simulink model "BatterySOHEstimation"  (R2024b)
settings: Solver=VariableStepAuto  StartTime=0.0  StopTime=3600  FixedStep=Ts  RelTol=1e-3  EnableMultiTasking=on
PreLoadFcn:
  | BatterySOHEstimationData;
values from neighbouring files (symbols this model uses):
  R = 0.05    [BatterySOHEstimationData.m]
  R00 = 0.008    [BatterySOHEstimationData.m]
  R0_mat = [.0117, .0085, .009; .011, .0085, .009;     .0114, .0087, .0092; .0107, .0082, .0088; .0107, .0083, .0091;     .0113, .0085, .0089; .0116, .0085, .0089]    [BatterySOHEstimationData.m]
  SOC0 = 0.65    [BatterySOHEstimationData.m]
  Ts = 1    [BatterySOHEstimationData.m]
undefined symbols (not defined in the file or in its folder): battery_builder_rtmsupport, gcbh
libraries: mBatteryPack_series_lib x414, mBatteryPack_lib x72, fl_lib x46, nesl_utility x22, BatteryEstimators x12, simulink x11, dspstat3 x9, PouchBatteryPack_lib x6, BatteryCurrentManagement x2, batteryecm_lib x1, SingleCellBatteryPack_lib x1
(part 1 of 26)
CloseFcn:
  | try
  |     close(h1_BatterySOHEstimation)
  | catch
  | end
  | 
  | clear h1_BatterySOHEstimation
  | 
  | clear BatterySOHEstimationSimlog
  | clear BatterySOHEstimationLogsout
  | 
  | clear AH SOC_vec T_vec R0_mat R1_mat tau1_mat
  | clear V0_mat Q R P0 initialSOC SOC0 R00 Ts
  | clear cell_area h_conv thermal_mass
Description:
  | Battery State-of-Health Estimation
settings Model: SimulationMode=accelerator  Creator=The MathWorks, Inc.  LastModifiedBy=marco
settings SolverCC: AlgebraicLoopSolver=TrustRegion  AutoInsertRateTranBlk=on  MaxZcPerStep=1
settings DataIOCC: MaxDataPoints=370000  ReturnWorkspaceOutputs=off  SignalLoggingName=BatterySOHEstimationLogsout
settings OptimizationCC: ReuseModelBlockBuffer=off  LifeSpan=inf
settings DebuggingCC: UnconnectedInputMsg=warning  UnconnectedOutputMsg=warning  UnconnectedLineMsg=warning  SFUnexpectedBacktrackingDiag=warning  SFNoUnconditionalDefaultTransitionDiag=warning  SFExecutionAtInitializationDiag=none  ArithmeticOperatorsInVariantConditions=warning
settings ModelReferenceCC: EnableRefExpFcnMdlSchedulingChecks=on
settings SFSimCC: SimUseLocalCustomCode=off  CustomCodeUndefinedFunction=UseInterfaceOnly
settings RTWCC: RTWUseLocalCustomCode=off  GPUComputeCapability=3.5  DLArmComputeVersion=19.05
settings CodeAppCC: StateflowObjectComments=on
settings GRTTargetCC: TargetLangStandard=C89/C90 (ANSI)
settings ConfigComp: CovMetricSettings=dw  CovSaveCumulativeToWorkspaceVar=on  CovSaveSingleToWorkspaceVar=on  CovExternalEMLEnable=off
settings SimscapeCC: SimscapeLogType=all  SimscapeLogSimulationStatistics=on  SimscapeLogName=BatterySOHEstimationSimlog  SimscapeLogDataHistory=370000

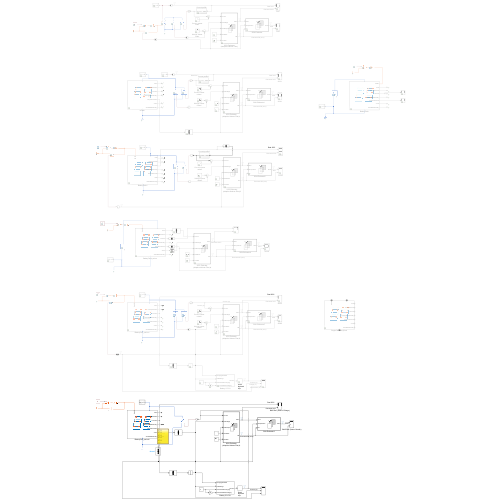
[thumbnail: Simulink's stored preview of the top-level diagram]
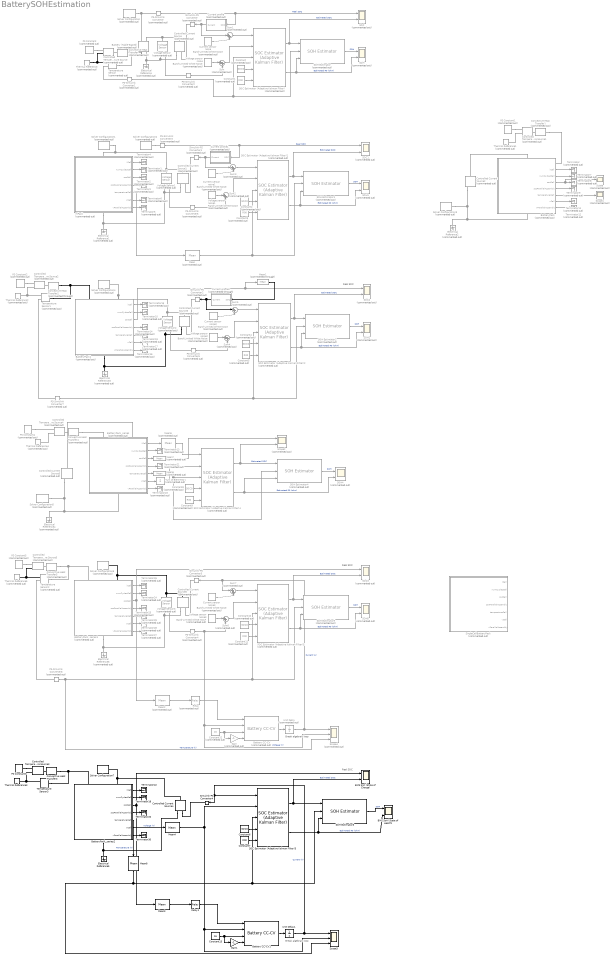
== system BatterySOHEstimation ==
  note: Real SOC
  note: Real SOC
  note: Break algebraic loop
  note: Real SOC
  note: Break algebraic loop
  BMS SoC (State of Charge) : Scope  NumInputPorts=2
  BMS SoH (State of Health) : Scope  NumInputPorts=2
  Battery (Table-Based) : batteryecm_lib/Battery (Table-Based)  Commented=on  SOC_vec=SOC_vec  T_dependence=simscape.enum.tablebattery.temperature_dependence.yes  prm_dir=simscape.enum.tablebattery.prm_dir.noCurrentDirectionality  T_vec=T_vec K  V0_mat=V0_mat V  V0_vec=[3.5057, 3.566, 3.6337, 3.7127, 3.9259, 4.0777, 4.1928] V  V_range=[0, inf] V  R0_mat=R0_mat Ohm  R0_vec=[.0085, .0085, .0087, .0082, .0083, .0085, .0085] Ohm  R0_dis_mat=[.0117, .0085, .009; .011, .0085, .009; .0114, .0087, .0092; .0107, .0082, .0088; .0107, .0083, .0091; .0113, .0085, .0089; .0116, .0085, .0089] Ohm  R0_dis_vec=[.0085, .0085, .0087, .0082, .0083, .0085, .0085] Ohm  R0_ch_mat=[.0117, .0085, .009; .011, .0085, .009; .0114, .0087, .0092; .0107, .0082, .0088; .0107, .0083, .0091; .0113, .0085, .0089; .0116, .0085, .0089] Ohm  R0_ch_vec=[.0085, .0085, .0087, .0082, .0083, .0085, .0085] Ohm  AH=AH A*hr  prm_leak=simscape.enum.tablebattery.prm_leak.disabled  Rleak_vec=[8000, 7000, 6000] Ohm  Rleak=7e3 Ohm  extrapolation_option=simscape.enum.extrapolation.nearest  SOC_port=simscape.enum.tablebattery.enable.yes  prm_dyn=simscape.enum.tablebattery.prm_dyn.rc1  R1_mat=R1_mat Ohm  R1_vec=[.0029, .0024, .0026, .0016, .0023, .0018, .0017] Ohm  tau1_mat=tau1_mat s  tau1_vec=[36, 45, 105, 29, 77, 33, 39] s  R2_mat=[.0109, .0029, .0013; .0069, .0024, .0012; .0047, .0026, .0013; .0034, .0016, .001; .0033, .0023, .0014; .0033, .0018, .0011; .0028, .0017, .0011] Ohm  R2_vec=[.0029, .0024, .0026, .0016, .0023, .0018, .0017] Ohm  tau2_mat=[20, 36, 39; 31, 45, 39; 109, 105, 61; 36, 29, 26; 59, 77, 67; 40, 33, 29; 25, 39, 33] s  tau2_vec=[36, 45, 105, 29, 77, 33, 39] s  R3_mat=[.0109, .0029, .0013; .0069, .0024, .0012; .0047, .0026, .0013; .0034, .0016, .001; .0033, .0023, .0014; .0033, .0018, .0011; .0028, .0017, .0011] Ohm  R3_vec=[.0029, .0024, .0026, .0016, .0023, .0018, .0017] Ohm  tau3_mat=[20, 36, 39; 31, 45, 39; 109, 105, 61; 36, 29, 26; 59, 77, 67; 40, 33, 29; 25, 39, 33] s  tau3_vec=[36, 45, 105, 29, 77, 33, 39] s  R4_mat=[.0109, .0029, .0013; .0069, .0024, .0012; .0047, .0026, .0013; .0034, .0016, .001; .0033, .0023, .0014; .0033, .0018, .0011; .0028, .0017, .0011] Ohm  R4_vec=[.0029, .0024, .0026, .0016, .0023, .0018, .0017] Ohm  tau4_mat=[20, 36, 39; 31, 45, 39; 109, 105, 61; 36, 29, 26; 59, 77, 67; 40, 33, 29; 25, 39, 33] s  tau4_vec=[36, 45, 105, 29, 77, 33, 39] s  R5_mat=[.0109, .0029, .0013; .0069, .0024, .0012; .0047, .0026, .0013; .0034, .0016, .001; .0033, .0023, .0014; .0033, .0018, .0011; .0028, .0017, .0011] Ohm  R5_vec=[.0029, .0024, .0026, .0016, .0023, .0018, .0017] Ohm  tau5_mat=[20, 36, 39; 31, 45, 39; 109, 105, 61; 36, 29, 26; 59, 77, 67; 40, 33, 29; 25, 39, 33] s  tau5_vec=[36, 45, 105, 29, 77, 33, 39] s  prm_fade=simscape.enum.tablebattery.prm_fade.equations  N0=10  dV0=0  dR0=100  dAH=0  dRleak=0  dR1=0  dR2=0  dR3=0  dR4=0  dR5=0  N0vec=[100, 200, 300]  Tfadevec=[298.15, 323.15] K  dV0vec=[0, 0, 0]  dR0vec=[0, 0, 0]  dAHvec=[0, 0, 0]  dRleakvec=[0, 0, 0]  dR1vec=[0, 0, 0]  dR2vec=[0, 0, 0]  dR3vec=[0, 0, 0]  dR4vec=[0, 0, 0]  dR5vec=[0, 0, 0]  dV0mat=[0, 0; 0, 0; 0, 0]  dR0mat=[0, 0; 0, 0; 0, 0]  dAHmat=[0, 0; 0, 0; 0, 0]  dRleakmat=[0, 0; 0, 0; 0, 0]  dR1mat=[0, 0; 0, 0; 0, 0]  dR2mat=[0, 0; 0, 0; 0, 0]  dR3mat=[0, 0; 0, 0; 0, 0]  dR4mat=[0, 0; 0, 0; 0, 0]  dR5mat=[0, 0; 0, 0; 0, 0]  prm_age_modeling=simscape.enum.tablebattery.prm_age_modeling.equation  storage_dt_age_vec=[0] d  storage_T_age_vec=[273] K  prm_age_OCV=simscape.enum.tablebattery.prm_age_OCV.OCV  OCV_age=0.9  SOC_age=0.6  prm_age_resistance=simscape.enum.tablebattery.prm_age.disabled  OCV_scaling_age_resistance=2.2134e6  OCV_offset_age_resistance=1.632e6  temp_exp_age_resistance=0.515833569 V  t_exp_age_resistance=0.75  T_age_vec_resistance=[273.15, 298.15, 323.15] K  dt_age_vec_resistance=[90, 180, 270, 360] d  dR0_age_vec=[0, 0, 0]  t_meas_dR0_age=100 d  dR0_age_mat=[0, 0, 0; 0, 0, 0; 0, 0, 0; 0, 0, 0]  prm_age_capacity=simscape.enum.tablebattery.prm_age.disabled  OCV_scaling_age_capacity=1.5097e07  OCV_offset_age_capacity=8.3625e06  temp_exp_age_capacity=0.6011 V  t_exp_age_capacity=0.75  T_age_vec_capacity=[273.15, 298.15, 323.15] K  dt_age_vec_capacity=[90, 180, 270, 360] d  dAH_age_vec=[0, 0, 0]  t_meas_dAH_age=100 d  dAH_age_mat=[0, 0, 0; 0, 0, 0; 0, 0, 0; 0, 0, 0]  thermal_port=simscape.enum.thermaleffects.model  temperature=298.15 K  thermal_mass=thermal_mass J/K  i_specify=off  i_priority=None  i=0 A  i_nominal_specify=off  i_nominal_value=1  i_nominal_unit=A  v_specify=off  v_priority=None  v=0 V  v_nominal_specify=off  v_nominal_value=1  v_nominal_unit=V  stateOfCharge_specify=on  stateOfCharge_priority=High  stateOfCharge=initialSOC  stateOfCharge_nominal_specify=off  stateOfCharge_nominal_value=1  stateOfCharge_nominal_unit=1  num_cycles_specify=off  num_cycles_priority=High  num_cycles=0  num_cycles_nominal_specify=off  num_cycles_nominal_value=1  num_cycles_nominal_unit=1  cell_temperature_specify=off  cell_temperature_priority=High  cell_temperature=293.15 K  cell_temperature_nominal_specify=off  cell_temperature_nominal_value=1  cell_temperature_nominal_unit=K
  Battery CC-CV : BatteryCurrentManagement/Battery CC-CV  Commented=on  MaxCellVoltage=3.8  Kp=0.25  Ki=0.01  Kaw=5  Kt=1  Ts=Ts
      settings: LibrarySourceBlock=batt_sl_lib/Current Management/Battery CC-CV
  Battery CC-CV1 : BatteryCurrentManagement/Battery CC-CV  MaxCellVoltage=3.8  Kp=0.45  Ki=0.01  Kaw=0  Kt=1  Ts=Ts
      settings: LibrarySourceBlock=batt_sl_lib/Current Management/Battery CC-CV
  BatteryPack : Subsystem  Commented=on  LoadFcn=battery_builder_rtmsupport('loadfcn',gcbh);
      settings: CopyFcn=battery_builder_rtmsupport('copyfcn',gcbh);  PreCopyFcn=battery_builder_rtmsupport('precopyfcn',gcbh);  PreDeleteFcn=battery_builder_rtmsupport('predeletefcn',gcbh);  PortSchema="{\"entries\":[{\"content\":{\"sides\":[{\"content\":{\"connectorIds\":[\"LConn1\"]},\"type\":\"ConnectorPlacement.EquallySpacedRectSide\",\"uuid\":\"7cd69c20-e5e1-4b8c-8ba2-b614cc84860a\"},{\"content\":{\"connectorIds\":[\"RConn1\"],\"side\":\"RIGHT\"},\"type\":\"ConnectorPlacement.EquallySpacedRectSide\",\"uuid\":\"49751c64-c6f5-4ea3-9cf1-2e6b12ee4ed0\"},{\"content\":{\"side\":\"TOP\"},\"type\":\"ConnectorPlacement.EquallySpacedRectSide\",\"uuid\":\"6273f34b-e7ea-45b8-b616-79ccc1698162\"},{\"content\":{\"connectorIds\":[\"RConn2\",\"Out1\",\"Out2\",\"Out3\",\"Out4\",\"Out5\",\"Out6\",\"Out7\"],\"side\":\"BOTTOM\"},\"type\":\"ConnectorPlacement.EquallySpacedRectSide\",\"uuid\":\"615cff9d-d28d-4c12-a58c-1414f05a82ef\"}]},\"type\":\"ConnectorPlacement.EquallySpacedConnector\",\"uuid\":\"c104401d-9cfe-42a1-b1e2-079ef8e2ed69\"}],\"packageUris\":[\"http://schema.mathworks.com/mf0/Connector/R2020b\"],\"version\":\"1.0\"}"
      mask Display: image('$imagefile')
  BatteryPack1 : Subsystem  Commented=on  LoadFcn=battery_builder_rtmsupport('loadfcn',gcbh);
      settings: CopyFcn=battery_builder_rtmsupport('copyfcn',gcbh);  PreCopyFcn=battery_builder_rtmsupport('precopyfcn',gcbh);  PreDeleteFcn=battery_builder_rtmsupport('predeletefcn',gcbh);  PortSchema="{\"entries\":[{\"content\":{\"sides\":[{\"content\":{\"connectorIds\":[\"LConn1\",\"LConn2\"]},\"type\":\"ConnectorPlacement.EquallySpacedRectSide\",\"uuid\":\"7cd69c20-e5e1-4b8c-8ba2-b614cc84860a\"},{\"content\":{\"connectorIds\":[\"RConn1\"],\"side\":\"RIGHT\"},\"type\":\"ConnectorPlacement.EquallySpacedRectSide\",\"uuid\":\"49751c64-c6f5-4ea3-9cf1-2e6b12ee4ed0\"},{\"content\":{\"side\":\"TOP\"},\"type\":\"ConnectorPlacement.EquallySpacedRectSide\",\"uuid\":\"6273f34b-e7ea-45b8-b616-79ccc1698162\"},{\"content\":{\"connectorIds\":[\"Out1\",\"Out2\",\"Out3\",\"Out4\",\"Out5\",\"Out6\",\"Out7\"],\"side\":\"BOTTOM\"},\"type\":\"ConnectorPlacement.EquallySpacedRectSide\",\"uuid\":\"615cff9d-d28d-4c12-a58c-1414f05a82ef\"}]},\"type\":\"ConnectorPlacement.EquallySpacedConnector\",\"uuid\":\"c104401d-9cfe-42a1-b1e2-079ef8e2ed69\"}],\"packageUris\":[\"http://schema.mathworks.com/mf0/Connector/R2020b\"],\"version\":\"1.0\"}"
      mask Display: image('$imagefile')
  BatteryPack_series : Subsystem  Commented=on  LoadFcn=battery_builder_rtmsupport('loadfcn',gcbh);
      settings: CopyFcn=battery_builder_rtmsupport('copyfcn',gcbh);  PreCopyFcn=battery_builder_rtmsupport('precopyfcn',gcbh);  PreDeleteFcn=battery_builder_rtmsupport('predeletefcn',gcbh);  PortSchema="{\"entries\":[{\"content\":{\"sides\":[{\"content\":{\"connectorIds\":[\"LConn1\",\"LConn2\"]},\"type\":\"ConnectorPlacement.EquallySpacedRectSide\",\"uuid\":\"25444e28-ed8a-4b61-b35e-6e8ef2c879d6\"},{\"content\":{\"connectorIds\":[\"RConn1\"],\"side\":\"RIGHT\"},\"type\":\"ConnectorPlacement.EquallySpacedRectSide\",\"uuid\":\"46764c24-5d85-4a00-a493-2df4d9019def\"},{\"content\":{\"side\":\"TOP\"},\"type\":\"ConnectorPlacement.EquallySpacedRectSide\",\"uuid\":\"3e1ac1ec-620a-4d1e-8b60-72c25ac46c33\"},{\"content\":{\"connectorIds\":[\"Out1\",\"Out2\",\"Out3\",\"Out4\",\"Out5\",\"Out6\",\"Out7\"],\"side\":\"BOTTOM\"},\"type\":\"ConnectorPlacement.EquallySpacedRectSide\",\"uuid\":\"68487603-14c8-46b3-8207-435891d1f14d\"}]},\"type\":\"ConnectorPlacement.EquallySpacedConnector\",\"uuid\":\"c9c2bba1-f437-4912-90d2-63acf03ea22d\"}],\"packageUris\":[\"http://schema.mathworks.com/mf0/Connector/R2020b\"],\"version\":\"1.0\"}"
      mask Display: image('$imagefile')
  BatteryPack_series1 : Subsystem  Commented=on  LoadFcn=battery_builder_rtmsupport('loadfcn',gcbh);
      settings: CopyFcn=battery_builder_rtmsupport('copyfcn',gcbh);  PreCopyFcn=battery_builder_rtmsupport('precopyfcn',gcbh);  PreDeleteFcn=battery_builder_rtmsupport('predeletefcn',gcbh);  PortSchema="{\"entries\":[{\"content\":{\"sides\":[{\"content\":{\"connectorIds\":[\"LConn1\",\"LConn2\"]},\"type\":\"ConnectorPlacement.EquallySpacedRectSide\",\"uuid\":\"25444e28-ed8a-4b61-b35e-6e8ef2c879d6\"},{\"content\":{\"connectorIds\":[\"RConn1\"],\"side\":\"RIGHT\"},\"type\":\"ConnectorPlacement.EquallySpacedRectSide\",\"uuid\":\"46764c24-5d85-4a00-a493-2df4d9019def\"},{\"content\":{\"side\":\"TOP\"},\"type\":\"ConnectorPlacement.EquallySpacedRectSide\",\"uuid\":\"3e1ac1ec-620a-4d1e-8b60-72c25ac46c33\"},{\"content\":{\"connectorIds\":[\"Out1\",\"Out2\",\"Out3\",\"Out4\",\"Out5\",\"Out6\",\"Out7\"],\"side\":\"BOTTOM\"},\"type\":\"ConnectorPlacement.EquallySpacedRectSide\",\"uuid\":\"68487603-14c8-46b3-8207-435891d1f14d\"}]},\"type\":\"ConnectorPlacement.EquallySpacedConnector\",\"uuid\":\"c9c2bba1-f437-4912-90d2-63acf03ea22d\"}],\"packageUris\":[\"http://schema.mathworks.com/mf0/Connector/R2020b\"],\"version\":\"1.0\"}"
      mask Display: image('$imagefile')
  BatteryPack_series2 : Subsystem  LoadFcn=battery_builder_rtmsupport('loadfcn',gcbh);
      settings: CopyFcn=battery_builder_rtmsupport('copyfcn',gcbh);  PreCopyFcn=battery_builder_rtmsupport('precopyfcn',gcbh);  PreDeleteFcn=battery_builder_rtmsupport('predeletefcn',gcbh);  PortSchema="{\"entries\":[{\"content\":{\"sides\":[{\"content\":{\"connectorIds\":[\"LConn1\",\"LConn2\"]},\"type\":\"ConnectorPlacement.EquallySpacedRectSide\",\"uuid\":\"25444e28-ed8a-4b61-b35e-6e8ef2c879d6\"},{\"content\":{\"connectorIds\":[\"RConn1\"],\"side\":\"RIGHT\"},\"type\":\"ConnectorPlacement.EquallySpacedRectSide\",\"uuid\":\"46764c24-5d85-4a00-a493-2df4d9019def\"},{\"content\":{\"side\":\"TOP\"},\"type\":\"ConnectorPlacement.EquallySpacedRectSide\",\"uuid\":\"3e1ac1ec-620a-4d1e-8b60-72c25ac46c33\"},{\"content\":{\"connectorIds\":[\"Out1\",\"Out2\",\"Out3\",\"Out4\",\"Out5\",\"Out6\",\"Out7\"],\"side\":\"BOTTOM\"},\"type\":\"ConnectorPlacement.EquallySpacedRectSide\",\"uuid\":\"68487603-14c8-46b3-8207-435891d1f14d\"}]},\"type\":\"ConnectorPlacement.EquallySpacedConnector\",\"uuid\":\"c9c2bba1-f437-4912-90d2-63acf03ea22d\"}],\"packageUris\":[\"http://schema.mathworks.com/mf0/Connector/R2020b\"],\"version\":\"1.0\"}"
      mask Display: image('$imagefile')
  Constant{,2,4,8,10} (5 alike) : Constant  Commented=on  Value=SOC0
  Constant{1,3,5,9,11} (5 alike) : Constant  Commented=on  Value=R00
  Constant12 : Constant  Commented=on  Value=15
  Constant13 : Constant  Value=15
  Constant6 : Constant  Value=SOC0
  Constant7 : Constant  Value=R00
  Controlled Temperature Source{,1..2,4..5} (5 alike) : fl_lib/Thermal/Thermal Sources/Controlled Temperature Source  Commented=on
  Controlled Temperature Source3 : fl_lib/Thermal/Thermal Sources/Controlled Temperature Source
  Controlled Current Source{,1..3,5..6} (6 alike) : fl_lib/Electrical/Electrical Sources/Controlled Current Source  Commented=on
  Controlled Current Source4 : fl_lib/Electrical/Electrical Sources/Controlled Current Source
  Convective Heat Transfer{,1,4..5} (4 alike) : fl_lib/Thermal/Thermal Elements/Convective Heat Transfer  Commented=on  thermal_type=foundation.enum.constant_variable.constant  area=0.1019 m^2  heat_tr_coeff=5 W/(K*m^2)  min_heat_tr_coeff=1e-3 W/(K*m^2)  T_specify=off  T_priority=None  T=0 K  T_nominal_specify=off  T_nominal_value=1  T_nominal_unit=K  Q_specify=off  Q_priority=None  Q=0 W  Q_nominal_specify=off  Q_nominal_value=1  Q_nominal_unit=W
  Convective Heat Transfer2 : fl_lib/Thermal/Thermal Elements/Convective Heat Transfer  Commented=through  thermal_type=foundation.enum.constant_variable.constant  area=0.1019 m^2  heat_tr_coeff=5 W/(K*m^2)  min_heat_tr_coeff=1e-3 W/(K*m^2)  T_specify=off  T_priority=None  T=0 K  T_nominal_specify=off  T_nominal_value=1  T_nominal_unit=K  Q_specify=off  Q_priority=None  Q=0 W  Q_nominal_specify=off  Q_nominal_value=1  Q_nominal_unit=W
  Convective Heat Transfer3 : fl_lib/Thermal/Thermal Elements/Convective Heat Transfer  thermal_type=foundation.enum.constant_variable.constant  area=0.1019 m^2  heat_tr_coeff=5 W/(K*m^2)  min_heat_tr_coeff=1e-3 W/(K*m^2)  T_specify=off  T_priority=None  T=0 K  T_nominal_specify=off  T_nominal_value=1  T_nominal_unit=K  Q_specify=off  Q_priority=None  Q=0 W  Q_nominal_specify=off  Q_nominal_value=1  Q_nominal_unit=W
  Current profile : Subsystem  Commented=on
  Current profile1 : Subsystem  Commented=on
  Current profile2 : Subsystem  Commented=through
  Current sensor noise{,1..3} (4 alike) : simulink/Sources/Band-Limited White Noise  Commented=on  Cov=1e-3  Ts=1  seed=1
  Electrical Reference{,1..4,6} (6 alike) : fl_lib/Electrical/Electrical Elements/Electrical Reference  Commented=on
  Electrical Reference5 : fl_lib/Electrical/Electrical Elements/Electrical Reference
  Gain : Gain  Commented=on  Gain=-1
  Gain1 : Gain  Gain=-1
  Mean{,2,5..7} (5 alike) : dspstat3/Mean  Commented=on  run=off  InputProcessing=Columns as channels (frame based)  reset_popup=None  directionMode=Each column  dimension=1  roiEnable=off  roiType=Rectangles  roiPortion=Entire ROI  roiOutput=Individual statistics for each ROI  roiFlag=off  roundingMode=Floor  overflowMode=off  outputDataTypeStr=Inherit: Same as accumulator  outputMin=[]  outputMax=[]  outputLastDataTypeStr=Inherit: Same as accumulator
  Mean1 : dspstat3/Mean  Commented=through  run=off  InputProcessing=Columns as channels (frame based)  reset_popup=None  directionMode=Each column  dimension=1  roiEnable=off  roiType=Rectangles  roiPortion=Entire ROI  roiOutput=Individual statistics for each ROI  roiFlag=off  roundingMode=Floor  overflowMode=off  outputDataTypeStr=Inherit: Same as accumulator  outputMin=[]  outputMax=[]  outputLastDataTypeStr=Inherit: Same as accumulator
  Mean3 : dspstat3/Mean  run=off  InputProcessing=Columns as channels (frame based)  reset_popup=None  directionMode=Each column  dimension=1  roiEnable=off  roiType=Rectangles  roiPortion=Entire ROI  roiOutput=Individual statistics for each ROI  roiFlag=off  roundingMode=Floor  overflowMode=off  outputDataTypeStr=Inherit: Same as accumulator  outputMin=[]  outputMax=[]  outputLastDataTypeStr=Inherit: Same as accumulator
  Mean4 : dspstat3/Mean  run=off  InputProcessing=Columns as channels (frame based)  reset_popup=None  directionMode=Each column  dimension=1  roiEnable=off  roiType=Rectangles  roiPortion=Entire ROI  roiOutput=Individual statistics for each ROI  roiFlag=off  roundingMode=Floor  overflowMode=off  outputDataTypeStr=Inherit: Same as accumulator  outputMin=[]  outputMax=[]  outputLastDataTypeStr=Inherit: Same as accumulator
  Mean8 : dspstat3/Mean  run=off  InputProcessing=Columns as channels (frame based)  reset_popup=None  directionMode=Each column  dimension=1  roiEnable=off  roiType=Rectangles  roiPortion=Entire ROI  roiOutput=Individual statistics for each ROI  roiFlag=off  roundingMode=Floor  overflowMode=off  outputDataTypeStr=Inherit: Same as accumulator  outputMin=[]  outputMax=[]  outputLastDataTypeStr=Inherit: Same as accumulator
  PS Constant{,1..2,4..5} (5 alike) : fl_lib/Physical Signals/Sources/PS Constant  Commented=on  constant=292.15 K
  PS Constant3 : fl_lib/Physical Signals/Sources/PS Constant  constant=423.15 K
  PS-Simulink Converter{,1..8} (9 alike) : nesl_utility/PS-Simulink Converter  Commented=on  PhysicalDomain=network_engine_domain  SubClassName=ps_output  LeftPortType=input  RightPortType=output  PseudoPeriodic=off  Frequencies=[]  VectorFormat=inherit  Unit=inherit  AffineConversion=off
  Relay : Relay  Commented=on  OnSwitchValue=0.9186  OffSwitchValue=0.3  OnOutputValue=0  OffOutputValue=1
  Relay1 : Relay  OnSwitchValue=0.9186  OffSwitchValue=0.3  OnOutputValue=0  OffOutputValue=1
  SOC{,1..3} (4 alike) : Scope  Commented=on  NumInputPorts=2
  SOC Estimator (Adaptive Kalman Filter) : BatteryEstimators/SOC Estimator (Adaptive Kalman Filter)  Commented=on  CurrentInputPartition=off  filterType=Unscented Kalman filter  alpha=1  beta=2  kappa=0  Q=Q  Q_2RC=|  R=R  P0=P0  P0_2RC="[1e-5 0 0 0; 0 1 0 0;0 0  1 0; 0 0 0 1e-5]"  Ts=Ts  chargeDynamics=One time-constant dynamics  SOC_vec=SOC_vec  T_vec=T_vec  R1_mat=R1_mat  tau1_mat=tau1_mat  R2_mat=[.0109, .0029, .0013; .0069, .0024, .0012; .0047, .0026, .0013; .0034, .0016, .001; .0033, .0023, .0014; .0033, .0018, .0011; .0028, .0017, .0011]  tau2_mat=[20, 36, 39; 31, 45, 39; 109, 105, 61; 36, 29, 26; 59, 77, 67; 40, 33, 29; 25, 39, 33]  V0_mat=V0_mat  AH=AH
      | [1e-6 0 0 0;
      | 0 1e-6 0 0;0 0 1e-6 0;0 0 0 1e-6]
  SOC Estimator (Adaptive Kalman Filter)1 : BatteryEstimators/SOC Estimator (Adaptive Kalman Filter)  Commented=on  CurrentInputPartition=off  filterType=Unscented Kalman filter  alpha=1  beta=2  kappa=0  Q=Q  Q_2RC=|  R=R  P0=P0  P0_2RC="[1e-5 0 0 0; 0 1 0 0;0 0  1 0; 0 0 0 1e-5]"  Ts=Ts  chargeDynamics=One time-constant dynamics  SOC_vec=SOC_vec  T_vec=T_vec  R1_mat=R1_mat  tau1_mat=tau1_mat  R2_mat=[.0109, .0029, .0013; .0069, .0024, .0012; .0047, .0026, .0013; .0034, .0016, .001; .0033, .0023, .0014; .0033, .0018, .0011; .0028, .0017, .0011]  tau2_mat=[20, 36, 39; 31, 45, 39; 109, 105, 61; 36, 29, 26; 59, 77, 67; 40, 33, 29; 25, 39, 33]  V0_mat=V0_mat  AH=AH
      | [1e-6 0 0 0;
      | 0 1e-6 0 0;0 0 1e-6 0;0 0 0 1e-6]
  SOC Estimator (Adaptive Kalman Filter)2 : BatteryEstimators/SOC Estimator (Adaptive Kalman Filter)  Commented=on  CurrentInputPartition=off  filterType=Unscented Kalman filter  alpha=1  beta=2  kappa=0  Q=Q  Q_2RC=|  R=R  P0=P0  P0_2RC="[1e-5 0 0 0; 0 1 0 0;0 0  1 0; 0 0 0 1e-5]"  Ts=Ts  chargeDynamics=One time-constant dynamics  SOC_vec=SOC_vec  T_vec=T_vec  R1_mat=R1_mat  tau1_mat=tau1_mat  R2_mat=[.0109, .0029, .0013; .0069, .0024, .0012; .0047, .0026, .0013; .0034, .0016, .001; .0033, .0023, .0014; .0033, .0018, .0011; .0028, .0017, .0011]  tau2_mat=[20, 36, 39; 31, 45, 39; 109, 105, 61; 36, 29, 26; 59, 77, 67; 40, 33, 29; 25, 39, 33]  V0_mat=V0_mat  AH=AH
      | [1e-6 0 0 0;
      | 0 1e-6 0 0;0 0 1e-6 0;0 0 0 1e-6]
  SOC Estimator (Adaptive Kalman Filter)3 : BatteryEstimators/SOC Estimator (Adaptive Kalman Filter)  CurrentInputPartition=on  filterType=Unscented Kalman filter  alpha=1  beta=2  kappa=0  Q=Q  Q_2RC=|  R=R  P0=P0  P0_2RC="[1e-5 0 0 0; 0 1 0 0;0 0  1 0; 0 0 0 1e-5]"  Ts=Ts  chargeDynamics=One time-constant dynamics  SOC_vec=SOC_vec  T_vec=T_vec  R1_mat=R1_mat  tau1_mat=tau1_mat  R2_mat=[.0109, .0029, .0013; .0069, .0024, .0012; .0047, .0026, .0013; .0034, .0016, .001; .0033, .0023, .0014; .0033, .0018, .0011; .0028, .0017, .0011]  tau2_mat=[20, 36, 39; 31, 45, 39; 109, 105, 61; 36, 29, 26; 59, 77, 67; 40, 33, 29; 25, 39, 33]  V0_mat=V0_mat  AH=AH
      | [1e-6 0 0 0;
      | 0 1e-6 0 0;0 0 1e-6 0;0 0 0 1e-6]
  SOC Estimator (Adaptive Kalman Filter)4 : BatteryEstimators/SOC Estimator (Adaptive Kalman Filter)  Commented=on  CurrentInputPartition=on  filterType=Unscented Kalman filter  alpha=1  beta=2  kappa=0  Q=Q  Q_2RC=|  R=R  P0=P0  P0_2RC="[1e-5 0 0 0; 0 1 0 0;0 0  1 0; 0 0 0 1e-5]"  Ts=Ts  chargeDynamics=One time-constant dynamics  SOC_vec=SOC_vec  T_vec=T_vec  R1_mat=R1_mat  tau1_mat=tau1_mat  R2_mat=[.0109, .0029, .0013; .0069, .0024, .0012; .0047, .0026, .0013; .0034, .0016, .001; .0033, .0023, .0014; .0033, .0018, .0011; .0028, .0017, .0011]  tau2_mat=[20, 36, 39; 31, 45, 39; 109, 105, 61; 36, 29, 26; 59, 77, 67; 40, 33, 29; 25, 39, 33]  V0_mat=V0_mat  AH=AH
      | [1e-6 0 0 0;
      | 0 1e-6 0 0;0 0 1e-6 0;0 0 0 1e-6]
  SOC Estimator (Adaptive Kalman Filter)5 : BatteryEstimators/SOC Estimator (Adaptive Kalman Filter)  Commented=on  CurrentInputPartition=on  filterType=Unscented Kalman filter  alpha=1  beta=2  kappa=0  Q=Q  Q_2RC=|  R=R  P0=P0  P0_2RC="[1e-5 0 0 0; 0 1 0 0;0 0  1 0; 0 0 0 1e-5]"  Ts=Ts  chargeDynamics=One time-constant dynamics  SOC_vec=SOC_vec  T_vec=T_vec  R1_mat=R1_mat  tau1_mat=tau1_mat  R2_mat=[.0109, .0029, .0013; .0069, .0024, .0012; .0047, .0026, .0013; .0034, .0016, .001; .0033, .0023, .0014; .0033, .0018, .0011; .0028, .0017, .0011]  tau2_mat=[20, 36, 39; 31, 45, 39; 109, 105, 61; 36, 29, 26; 59, 77, 67; 40, 33, 29; 25, 39, 33]  V0_mat=V0_mat  AH=AH
      | [1e-6 0 0 0;
      | 0 1e-6 0 0;0 0 1e-6 0;0 0 0 1e-6]
  SOH{,1..2,4..5} (5 alike) : Scope  Commented=on  NumInputPorts=2
  SOH Estimator{,1..2,4..5} (5 alike) : BatteryEstimators/SOH Estimator  Commented=on  SOC_vec=SOC_vec  T_vec=T_vec  R0_new_mat=R0_mat  R0_EOL_mat=R0_mat*3
  SOH Estimator3 : BatteryEstimators/SOH Estimator  SOC_vec=SOC_vec  T_vec=T_vec  R0_new_mat=R0_mat  R0_EOL_mat=R0_mat*3
  Scope : Scope  Commented=on
  Scope1 : Scope  Commented=on
  Scope2 : Scope  Commented=on  NumInputPorts=2
  Scope3 : Scope  NumInputPorts=3
  Scope4 : Scope  Commented=on  NumInputPorts=3
  Simulink-PS Converter{,1..3} (4 alike) : nesl_utility/Simulink-PS Converter  Commented=on  PhysicalDomain=network_engine_domain  SubClassName=ps_input  LeftPortType=input  RightPortType=output  PseudoPeriodic=off  Frequencies=[]  NoiseDistribution=none  NoiseParameters=[]  Unit=1  AffineConversion=off  FilteringAndDerivatives=provide  SimscapeFilterOrder=1  InputFilterTimeConstant=0.001  UdotUserProvided=0
  Simulink-PS Converter4 : nesl_utility/Simulink-PS Converter  PhysicalDomain=network_engine_domain  SubClassName=ps_input  LeftPortType=input  RightPortType=output  PseudoPeriodic=off  Frequencies=[]  NoiseDistribution=none  NoiseParameters=[]  Unit=1  AffineConversion=off  FilteringAndDerivatives=provide  SimscapeFilterOrder=1  InputFilterTimeConstant=0.001  UdotUserProvided=0
  SingleCellBatteryPack : Subsystem  Commented=on  LoadFcn=battery_builder_rtmsupport('loadfcn',gcbh);
      settings: CopyFcn=battery_builder_rtmsupport('copyfcn',gcbh);  PreCopyFcn=battery_builder_rtmsupport('precopyfcn',gcbh);  PreDeleteFcn=battery_builder_rtmsupport('predeletefcn',gcbh);  PortSchema="{\"entries\":[{\"content\":{\"sides\":[{\"content\":{\"connectorIds\":[\"LConn1\",\"LConn2\"]},\"type\":\"ConnectorPlacement.EquallySpacedRectSide\",\"uuid\":\"b37d56bf-7bdd-45ac-bd3e-9966f4ef20bd\"},{\"content\":{\"connectorIds\":[\"RConn1\"],\"side\":\"RIGHT\"},\"type\":\"ConnectorPlacement.EquallySpacedRectSide\",\"uuid\":\"5abecaa2-92ef-4380-bbec-04b1245a8d22\"},{\"content\":{\"side\":\"TOP\"},\"type\":\"ConnectorPlacement.EquallySpacedRectSide\",\"uuid\":\"215bade3-2994-41b1-8b89-4b38961bed55\"},{\"content\":{\"connectorIds\":[\"Out1\",\"Out2\",\"Out3\",\"Out4\",\"Out5\",\"Out6\",\"Out7\"],\"side\":\"BOTTOM\"},\"type\":\"ConnectorPlacement.EquallySpacedRectSide\",\"uuid\":\"a13df2c7-5e58-4639-a658-182c338bba4b\"}]},\"type\":\"ConnectorPlacement.EquallySpacedConnector\",\"uuid\":\"c07c30bf-c70d-4b4b-a0d3-a2a4bd58775b\"}],\"packageUris\":[\"http://schema.mathworks.com/mf0/Connector/R2020b\"],\"version\":\"1.0\"}"
      mask Display: image('$imagefile')
  Solver Configuration{,1..6} (7 alike) : nesl_utility/Solver Configuration  Commented=on  PhysicalDomain=network_engine_domain  SubClassName=solver  LeftPortType=input  RightPortType=generic  Tones=[]  Harmonics=[]  SimulateNoise=off  Profile=off  UseLocalSampling=off  EnableSwitchedLinearOptims=on  FrequencyDomain=off  UseCCode=off  RelTol=0.001  AbsTol=0.001  MinStep=1e-09  ToWorkspace=off  RevertToSquareIcSolve=off  NumHomotopyIterations=100  PhasorMode=off  PhasorModeNumHarmonics=1  ConsistencySolver=NEWTON_XTOL_AFTER_FTOL  IndexReductionMethod=DerivativeReplacement  DoDC=off  ResidualTolerance=1e-09  ConsistencyTolSource=GLOBAL  ConsistencyAbsTol=0.001  ConsistencyRelTol=0.001  ConsistencyTolFactor=0.001  UseLocalSolver=off  LocalSolverChoice=NE_BACKWARD_EULER_ADVANCER  ResolveIndetEquations=on  FunctionEvalNumThread=1  LocalSolverSampleTime=0.001  DoFixedCost=off  MaxNonlinIter=3  MaxModeIter=2  ComputeImpulses=off  ImpulseIterations=2  LinearAlgebra=auto  LinearAlgebraNumThread=0  EquationFormulation=NE_TIME_EF  DelaysMemoryBudget=1024  AutomaticFiltering=on  FilteringTimeConstant=0.001  PartitionStorageMethod=AS_NEEDED  PartitionMemoryBudget=1024  PartitionMethod=ROBUST  MultibodyUseLocalSolver=off  MultibodyLocalSolverChoice=ODE1  MultibodyLocalSolverSampleTime=0.001
  Solver Configuration7 : nesl_utility/Solver Configuration  PhysicalDomain=network_engine_domain  SubClassName=solver  LeftPortType=input  RightPortType=generic  Tones=[]  Harmonics=[]  SimulateNoise=off  Profile=off  UseLocalSampling=off  EnableSwitchedLinearOptims=on  FrequencyDomain=off  UseCCode=off  RelTol=0.001  AbsTol=0.001  MinStep=1e-09  ToWorkspace=off  RevertToSquareIcSolve=off  NumHomotopyIterations=100  PhasorMode=off  PhasorModeNumHarmonics=1  ConsistencySolver=NEWTON_XTOL_AFTER_FTOL  IndexReductionMethod=DerivativeReplacement  DoDC=off  ResidualTolerance=1e-09  ConsistencyTolSource=GLOBAL  ConsistencyAbsTol=0.001  ConsistencyRelTol=0.001  ConsistencyTolFactor=0.001  UseLocalSolver=off  LocalSolverChoice=NE_BACKWARD_EULER_ADVANCER  ResolveIndetEquations=on  FunctionEvalNumThread=1  LocalSolverSampleTime=0.001  DoFixedCost=off  MaxNonlinIter=3  MaxModeIter=2  ComputeImpulses=off  ImpulseIterations=2  LinearAlgebra=auto  LinearAlgebraNumThread=0  EquationFormulation=NE_TIME_EF  DelaysMemoryBudget=1024  AutomaticFiltering=on  FilteringTimeConstant=0.001  PartitionStorageMethod=AS_NEEDED  PartitionMemoryBudget=1024  PartitionMethod=ROBUST  MultibodyUseLocalSolver=off  MultibodyLocalSolverChoice=ODE1  MultibodyLocalSolverSampleTime=0.001
  Sum{,1..7} (8 alike) : Sum  Commented=on  Inputs=|++
  Sum of Elements1 : Sum  Commented=on  Inputs=+
  Temperature Sensor : fl_lib/Thermal/Thermal Sensors/Temperature Sensor  Commented=on  temperature_measure=foundation.enum.MeasurementReference.difference
  Temperature Sensor1 : fl_lib/Thermal/Thermal Sensors/Temperature Sensor  Commented=on  temperature_measure=foundation.enum.MeasurementReference.difference
  Temperature Sensor2 : fl_lib/Thermal/Thermal Sensors/Temperature Sensor  Commented=on  temperature_measure=foundation.enum.MeasurementReference.difference
  Temperature Sensor3 : fl_lib/Thermal/Thermal Sensors/Temperature Sensor  temperature_measure=foundation.enum.MeasurementReference.difference
  Terminator{,1..17,19,21,23..29} (27 alike) : Terminator  Commented=on
  Terminator{18,20,22,30} (4 alike) : Terminator
  Thermal Reference{,1..2,4..5} (5 alike) : fl_lib/Thermal/Thermal Elements/Thermal Reference  Commented=on
  Thermal Reference3 : fl_lib/Thermal/Thermal Elements/Thermal Reference
  Unit Delay : UnitDelay  Commented=on  SampleTime=-1  HasFrameUpgradeWarning=on
  Unit Delay1 : UnitDelay  SampleTime=-1  HasFrameUpgradeWarning=on
  Voltage Sensor{,1..3} (4 alike) : fl_lib/Electrical/Electrical Sensors/Voltage Sensor  Commented=on
  Voltage sensor noise{,1..3} (4 alike) : simulink/Sources/Band-Limited White Noise  Commented=on  Cov=1e-3  Ts=1  seed=23341
  mPack : Subsystem  Commented=on  LoadFcn=battery_builder_rtmsupport('loadfcn',gcbh);
      settings: CopyFcn=battery_builder_rtmsupport('copyfcn',gcbh);  PreCopyFcn=battery_builder_rtmsupport('precopyfcn',gcbh);  PreDeleteFcn=battery_builder_rtmsupport('predeletefcn',gcbh);  PortSchema="{\"entries\":[{\"content\":{\"sides\":[{\"content\":{\"connectorIds\":[\"LConn1\"]},\"type\":\"ConnectorPlacement.EquallySpacedRectSide\",\"uuid\":\"18ac6db1-889f-4c13-abdf-68c5c706792f\"},{\"content\":{\"connectorIds\":[\"RConn1\"],\"side\":\"RIGHT\"},\"type\":\"ConnectorPlacement.EquallySpacedRectSide\",\"uuid\":\"b261584e-a342-463c-abe3-25d391249932\"},{\"content\":{\"side\":\"TOP\"},\"type\":\"ConnectorPlacement.EquallySpacedRectSide\",\"uuid\":\"1e2a4c05-8071-4309-8496-9476190898ec\"},{\"content\":{\"connectorIds\":[\"Out1\",\"Out2\",\"Out3\",\"Out4\",\"Out5\",\"Out6\",\"Out7\"],\"side\":\"BOTTOM\"},\"type\":\"ConnectorPlacement.EquallySpacedRectSide\",\"uuid\":\"f9861d4f-af67-4d90-9e06-ff4308f00af4\"}]},\"type\":\"ConnectorPlacement.EquallySpacedConnector\",\"uuid\":\"f932596e-c7b7-41e5-b5ce-37463633e4ff\"}],\"packageUris\":[\"http://schema.mathworks.com/mf0/Connector/R2020b\"],\"version\":\"1.0\"}"
      mask Display: image('$imagefile')
  wires:
  PS-Simulink Converter2/1 -> Sum/2
  Sum1/1 -> SOC Estimator (Adaptive Kalman Filter)/1
  Sum/1 -> SOC Estimator (Adaptive Kalman Filter)/2
  PS-Simulink Converter1/1 -> SOH Estimator/2, SOC Estimator (Adaptive Kalman Filter)/3
  Constant/1 -> SOC Estimator (Adaptive Kalman Filter)/4
  Constant1/1 -> SOC Estimator (Adaptive Kalman Filter)/5
  SOC Estimator (Adaptive Kalman Filter)/1 -> SOH Estimator/1, SOC/2  "Estimated SOC"
  SOC Estimator (Adaptive Kalman Filter)/2 -> SOH/2, SOH Estimator/3  "Estimated R0 (ohm)"
  Current profile/1(Current) -> Sum1/1, Simulink-PS Converter/1
  PS-Simulink Converter/1 -> Current profile/1(SOC), SOC/1  "Real SOC"
  SOH Estimator/1 -> SOH/1  "SOH"
  Voltage sensor noise/1 -> Sum/1
  Current sensor noise/1 -> Sum1/2
  PS-Simulink Converter5/1 -> Sum2/2
  Sum3/1 -> SOC Estimator (Adaptive Kalman Filter)1/1
  Constant2/1 -> SOC Estimator (Adaptive Kalman Filter)1/4
  SOC Estimator (Adaptive Kalman Filter)1/1 -> SOH Estimator1/1, SOC1/2  "Estimated SOC"
  SOH Estimator1/1 -> SOH1/1  "SOH"
  Voltage sensor noise1/1 -> Sum2/1
  Sum2/1 -> SOC Estimator (Adaptive Kalman Filter)1/2
  Constant3/1 -> SOC Estimator (Adaptive Kalman Filter)1/5
  Current sensor noise1/1 -> Sum3/2
  PS-Simulink Converter3/1 -> Current profile1/1(SOC), SOC1/1  "Real SOC"
  Current profile1/1(Current) -> Sum3/1, Simulink-PS Converter1/1
  SOC Estimator (Adaptive Kalman Filter)1/2 -> SOH1/2, SOH Estimator1/3  "Estimated R0 (ohm)"
  mPack/7(vParallelAssembly) -> Terminator5/1
  mPack/4(socParallelAssembly) -> Terminator3/1
  mPack/3(socCell) -> Terminator2/1
  mPack/2(numCyclesCell) -> Terminator1/1
  mPack/6(vCell) -> Terminator6/1
  mPack/1(iCell) -> Terminator4/1
  mPack/5(temperatureCell) -> Mean/1
  Mean/1 -> SOC Estimator (Adaptive Kalman Filter)1/3, SOH Estimator1/2
  BatteryPack/1(iCell) -> Terminator/1
  BatteryPack/2(numCyclesCell) -> Terminator7/1
  BatteryPack/3(socCell) -> Scope/1, Terminator8/1
  BatteryPack/4(socParallelAssembly) -> Terminator9/1
  BatteryPack/5(temperatureCell) -> Scope1/1
  BatteryPack/6(vCell) -> Terminator11/1
  BatteryPack/7(vParallelAssembly) -> Terminator12/1
  PS-Simulink Converter7/1 -> SOC Estimator (Adaptive Kalman Filter)2/3, SOH Estimator2/2
  PS-Simulink Converter6/1 -> Sum4/2
  Sum5/1 -> SOC Estimator (Adaptive Kalman Filter)2/1
  SOC Estimator (Adaptive Kalman Filter)2/2 -> SOH2/2, SOH Estimator2/3  "Estimated R0 (ohm)"
  Current profile2/1(Current) -> Sum5/1, Simulink-PS Converter2/1
  Constant5/1 -> SOC Estimator (Adaptive Kalman Filter)2/5
  Current sensor noise2/1 -> Sum5/2
  BatteryPack1/6(vCell) -> Terminator17/1
  Sum4/1 -> SOC Estimator (Adaptive Kalman Filter)2/2
  SOH Estimator2/1 -> SOH2/1  "SOH"
  Constant4/1 -> SOC Estimator (Adaptive Kalman Filter)2/4
  SOC Estimator (Adaptive Kalman Filter)2/1 -> SOH Estimator2/1, SOC2/2  "Estimated SOC"
  Voltage sensor noise2/1 -> Sum4/1
  BatteryPack1/7(vParallelAssembly) -> Terminator16/1
  BatteryPack1/4(socParallelAssembly) -> Terminator14/1
  BatteryPack1/3(socCell) -> Mean1/1, SOC2/1
  BatteryPack1/2(numCyclesCell) -> Terminator10/1
  BatteryPack1/1(iCell) -> Terminator15/1
  BatteryPack1/5(temperatureCell) -> Terminator19/1
  Mean1/1 -> Current profile2/1(SOC)
  Mean5/1 -> SOC Estimator (Adaptive Kalman Filter)4/1
  BatteryPack_series/4(socParallelAssembly) -> Terminator21/1
  BatteryPack_series/7(vParallelAssembly) -> Terminator23/1
  BatteryPack_series/5(temperatureCell) -> Mean6/1
  Mean6/1 -> SOH Estimator4/2, SOC Estimator (Adaptive Kalman Filter)4/3
  Constant8/1 -> SOC Estimator (Adaptive Kalman Filter)4/4
  SOC Estimator (Adaptive Kalman Filter)4/1 -> SOH Estimator4/1, Scope2/2  "Estimated SOC"
  BatteryPack_series/6(vCell) -> Sum of Elements1/1
  BatteryPack_series/2(numCyclesCell) -> Terminator13/1
  Constant9/1 -> SOC Estimator (Adaptive Kalman Filter)4/5
  SOH Estimator4/1 -> SOH4/1  "SOH"
  Mean7/1 -> Scope2/1
  Sum of Elements1/1 -> SOC Estimator (Adaptive Kalman Filter)4/2
  SOC Estimator (Adaptive Kalman Filter)4/2 -> SOH Estimator4/3, SOH4/2  "Estimated R0 (ohm)"
  BatteryPack_series/1(iCell) -> Mean5/1
  BatteryPack_series/3(socCell) -> Mean7/1
  BatteryPack_series1/4(socParallelAssembly) -> Terminator25/1
  Sum6/1 -> SOC Estimator (Adaptive Kalman Filter)5/2
  SOC Estimator (Adaptive Kalman Filter)5/2 -> SOH5/2, SOH Estimator5/3  "Estimated R0 (ohm)"
  Voltage sensor noise3/1 -> Sum6/1
  Current sensor noise3/1 -> Sum7/2
  BatteryPack_series1/7(vParallelAssembly) -> Terminator27/1
  Sum7/1 -> SOC Estimator (Adaptive Kalman Filter)5/1
  BatteryPack_series1/2(numCyclesCell) -> Terminator24/1
  BatteryPack_series1/5(temperatureCell) -> Terminator29/1
  Constant10/1 -> SOC Estimator (Adaptive Kalman Filter)5/4
  SOC Estimator (Adaptive Kalman Filter)5/1 -> SOH Estimator5/1, SOC3/2  "Estimated SOC"
  SOH Estimator5/1 -> SOH5/1  "SOH"
  BatteryPack_series1/6(vCell) -> Terminator28/1
  BatteryPack_series1/1(iCell) -> Terminator26/1
  Constant11/1 -> SOC Estimator (Adaptive Kalman Filter)5/5
  Gain/1 -> Battery CC-CV/4
  Battery CC-CV/1 -> Unit Delay/1
  Relay/1 -> Battery CC-CV/1
  PS-Simulink Converter4/1 -> Sum6/2, Scope4/2, Battery CC-CV/2  "Voltage (V)"
  PS-Simulink Converter8/1 -> Scope4/3, SOC Estimator (Adaptive Kalman Filter)5/3, SOH Estimator5/2  "Temperature (K)"
  Unit Delay/1 -> Sum7/1, Simulink-PS Converter3/1, Scope4/1  "Current (A)"
  Constant12/1 -> Battery CC-CV/3, Gain/1
  BatteryPack_series1/3(socCell) -> Mean2/1, SOC3/1
  Mean2/1 -> Relay/1
  BatteryPack_series2/2(numCyclesCell) -> Terminator18/1
  SOH Estimator3/1 -> BMS SoH (State of Health)/1  "SOH"
  Constant6/1 -> SOC Estimator (Adaptive Kalman Filter)3/4
  Gain1/1 -> Battery CC-CV1/4
  BatteryPack_series2/3(socCell) -> Mean3/1, BMS SoC (State of Charge)/1
  Unit Delay1/1 -> Simulink-PS Converter4/1, SOC Estimator (Adaptive Kalman Filter)3/1, Scope3/1  "Current (A)"
  Mean3/1 -> Relay1/1
  Constant13/1 -> Battery CC-CV1/3, Gain1/1
  Battery CC-CV1/1 -> Unit Delay1/1
  BatteryPack_series2/6(vCell) -> Mean4/1  "Voltage (V)"
  SOC Estimator (Adaptive Kalman Filter)3/1 -> SOH Estimator3/1, BMS SoC (State of Charge)/2  "Estimated SOC"
  BatteryPack_series2/5(temperatureCell) -> Mean8/1  "Temperature (K)"
  Relay1/1 -> Battery CC-CV1/1
  BatteryPack_series2/1(iCell) -> Terminator22/1
  BatteryPack_series2/4(socParallelAssembly) -> Terminator20/1
  SOC Estimator (Adaptive Kalman Filter)3/2 -> SOH Estimator3/3, BMS SoH (State of Health)/2  "Estimated R0 (ohm)"
  BatteryPack_series2/7(vParallelAssembly) -> Terminator30/1
  Constant7/1 -> SOC Estimator (Adaptive Kalman Filter)3/5
  Mean4/1 -> Scope3/2, Battery CC-CV1/2, SOC Estimator (Adaptive Kalman Filter)3/2
  Mean8/1 -> SOC Estimator (Adaptive Kalman Filter)3/3, SOH Estimator3/2, Scope3/3
  connections:
  PS-Simulink Converter/LConn1 -- Battery (Table-Based)/LConn2 -- Solver Configuration/RConn1
  Electrical Reference/LConn1 -- Battery (Table-Based)/RConn1 -- Controlled Current Source/RConn2 -- Voltage Sensor/RConn2
  Voltage Sensor/LConn1 -- Battery (Table-Based)/LConn1 -- Controlled Current Source/LConn1
  Simulink-PS Converter/RConn1 -- Controlled Current Source/RConn1
  Voltage Sensor/RConn1 -- PS-Simulink Converter2/LConn1
  Temperature Sensor/LConn1 -- Battery (Table-Based)/RConn2 -- Convective Heat Transfer/LConn1
  Temperature Sensor/RConn1 -- Thermal Reference/LConn1 -- Controlled Temperature Source/RConn2
  Controlled Temperature Source/LConn1 -- Convective Heat Transfer/RConn1
  PS-Simulink Converter1/LConn1 -- Temperature Sensor/RConn2
  PS Constant/RConn1 -- Controlled Temperature Source/RConn1
  Voltage Sensor1/RConn2 -- Controlled Current Source1/RConn2 -- mPack/RConn1 -- Electrical Reference1/LConn1
  Controlled Current Source1/LConn1 -- mPack/LConn1 -- Solver Configuration1/RConn1 -- Voltage Sensor1/LConn1
  Simulink-PS Converter1/RConn1 -- Controlled Current Source1/RConn1
  PS-Simulink Converter5/LConn1 -- Voltage Sensor1/RConn1
  Solver Configuration2/RConn1 -- PS-Simulink Converter3/LConn1
  Controlled Current Source2/LConn1 -- BatteryPack/LConn1
  Controlled Current Source2/RConn2 -- Solver Configuration3/RConn1 -- BatteryPack/RConn1 -- Electrical Reference2/LConn1
  Convective Heat Transfer1/LConn1 -- BatteryPack/RConn2
  Controlled Temperature Source1/RConn2 -- Thermal Reference1/LConn1
  PS Constant1/RConn1 -- Controlled Temperature Source1/RConn1
  Controlled Temperature Source1/LConn1 -- Convective Heat Transfer1/RConn1
  Controlled Current Source3/LConn1 -- BatteryPack1/LConn2 -- Solver Configuration4/RConn1 -- Voltage Sensor2/LConn1
  Electrical Reference3/LConn1 -- BatteryPack1/RConn1 -- Controlled Current Source3/RConn2 -- Voltage Sensor2/RConn2
  PS-Simulink Converter6/LConn1 -- Voltage Sensor2/RConn1
  Simulink-PS Converter2/RConn1 -- Controlled Current Source3/RConn1
  PS Constant2/RConn1 -- Controlled Temperature Source2/RConn1
  Controlled Temperature Source2/RConn2 -- Temperature Sensor1/RConn1 -- Thermal Reference2/LConn1
  Controlled Temperature Source2/LConn1 -- Convective Heat Transfer2/RConn1
  Convective Heat Transfer2/LConn1 -- Temperature Sensor1/LConn1 -- BatteryPack1/LConn1
  PS-Simulink Converter7/LConn1 -- Temperature Sensor1/RConn2
  Controlled Current Source5/RConn2 -- Solver Configuration5/RConn1 -- Electrical Reference4/LConn1 -- BatteryPack_series/RConn1
  PS Constant4/RConn1 -- Controlled Temperature Source4/RConn1
  Controlled Temperature Source4/RConn2 -- Thermal Reference4/LConn1
  Controlled Temperature Source4/LConn1 -- Convective Heat Transfer4/RConn1
  Controlled Current Source5/LConn1 -- BatteryPack_series/LConn2
  Convective Heat Transfer4/LConn1 -- BatteryPack_series/LConn1
  Temperature Sensor2/LConn1 -- BatteryPack_series1/LConn1 -- Convective Heat Transfer5/LConn1
  Voltage Sensor3/LConn1 -- BatteryPack_series1/LConn2 -- Solver Configuration6/RConn1 -- Controlled Current Source6/LConn1
  Voltage Sensor3/RConn2 -- Controlled Current Source6/RConn2 -- BatteryPack_series1/RConn1 -- Electrical Reference6/LConn1
  Thermal Reference5/LConn1 -- Controlled Temperature Source5/RConn2 -- Temperature Sensor2/RConn1
  PS-Simulink Converter8/LConn1 -- Temperature Sensor2/RConn2
  PS Constant5/RConn1 -- Controlled Temperature Source5/RConn1
  PS-Simulink Converter4/LConn1 -- Voltage Sensor3/RConn1
  Controlled Temperature Source5/LConn1 -- Convective Heat Transfer5/RConn1
  Simulink-PS Converter3/RConn1 -- Controlled Current Source6/RConn1
  Controlled Current Source4/RConn2 -- Electrical Reference5/LConn1 -- BatteryPack_series2/RConn1
  Temperature Sensor3/RConn1 -- Thermal Reference3/LConn1 -- Controlled Temperature Source3/RConn2
  Convective Heat Transfer3/LConn1 -- Temperature Sensor3/LConn1 -- BatteryPack_series2/LConn1
  PS Constant3/RConn1 -- Controlled Temperature Source3/RConn1
  Controlled Temperature Source3/LConn1 -- Convective Heat Transfer3/RConn1
  Controlled Current Source4/RConn1 -- Simulink-PS Converter4/RConn1
  Controlled Current Source4/LConn1 -- Solver Configuration7/RConn1 -- BatteryPack_series2/LConn2
